simulink model "cl_e_5x"  (Simulink 7.4)
settings: Solver=ode15s  StartTime=0.0  StopTime=inf  MaxStep=5e-9  RelTol=1e-5
PreLoadFcn:
  | f=3.9e6; Cp=3.6e-9; Cx=3e-9;
undefined symbols (not defined in the file or in its folder): One, sided
libraries: powerlib x16, simulink x1, dspsnks4 x1, dsparch4 x1
settings Model: Creator=dbenson  LastModifiedBy=Dick
settings DataIOCC: SaveOutput=off  SaveTime=off  SignalLoggingName=sigsOut
settings OptimizationCC: BooleanDataType=off  InlineInvariantSignals=on  InitFltsAndDblsToZero=on
settings DebuggingCC: SaveWithParameterizedLinksMsg=none  SignalResolutionControl=TryResolveAllWithWarning  SolverPrmCheckMsg=none  MultiTaskDSMMsg=warning  MultiTaskCondExecSysMsg=none  StrictBusMsg=None
settings HardwareCC: TargetUnknown=on
settings RTWCC: IncludeERTFirstTime=on
settings GRTTargetCC: TargetFcnLib=ansi_tfl_tmw.mat

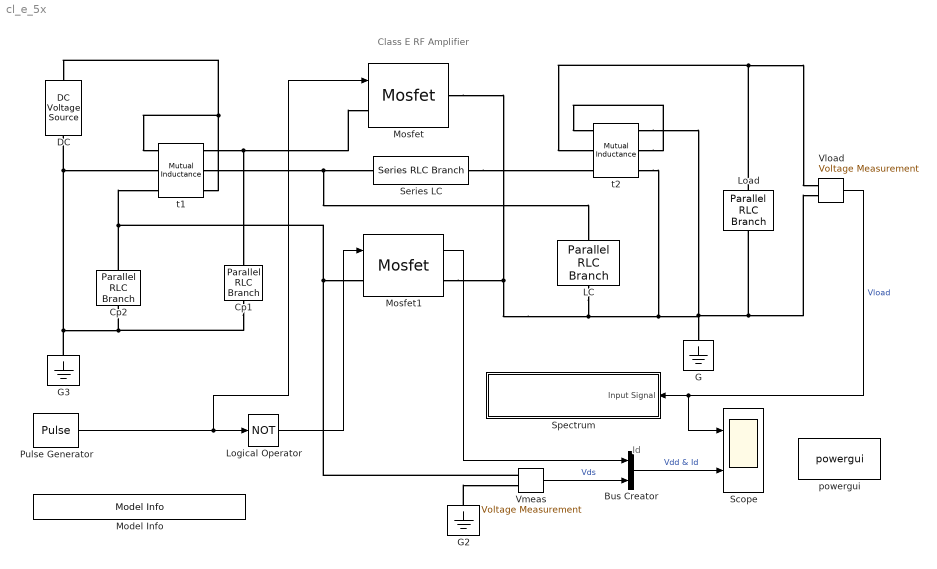
== system cl_e_5x ==
  note: Id
  note: Class E RF Amplifier
  Bus Creator : BusCreator  Inputs=2
  Cp1 : powerlib/Elements/Parallel RLC Branch  DialogController=POWERSYS.PowerSysDialog  PhysicalDomain=powersysdomain  SubClassName=unknown  LeftPortType=p1  RightPortType=p1  LConnTagsString=a  RConnTagsString=__new0  BranchType=C  Resistance=1.0  Inductance=1.0  SetiL0=off  InitialCurrent=0  Capacitance=Cp  Setx0=off  InitialVoltage=0  Measurements=None
  Cp2 : powerlib/Elements/Parallel RLC Branch  DialogController=POWERSYS.PowerSysDialog  PhysicalDomain=powersysdomain  SubClassName=unknown  LeftPortType=p1  RightPortType=p1  LConnTagsString=a  RConnTagsString=__new0  BranchType=C  Resistance=1.0  Inductance=1.0  SetiL0=off  InitialCurrent=0  Capacitance=Cp  Setx0=off  InitialVoltage=0  Measurements=None
  DC : powerlib/Electrical Sources/DC Voltage Source  Description=source block  DialogController=POWERSYS.PowerSysDialog  SystemSampleTime=-1  Amplitude=25  Measurements=None
      settings: AttributesFormatString=\n
  G : powerlib/Elements/Ground  DialogController=POWERSYS.PowerSysDialog  PhysicalDomain=powersysdomain  SubClassName=unknown  LeftPortType=p1  RightPortType=p1  LConnTagsString=a
  G2 : powerlib/Elements/Ground  DialogController=POWERSYS.PowerSysDialog  PhysicalDomain=powersysdomain  SubClassName=unknown  LeftPortType=p1  RightPortType=p1  LConnTagsString=a
  G3 : powerlib/Elements/Ground  DialogController=POWERSYS.PowerSysDialog  PhysicalDomain=powersysdomain  SubClassName=unknown  LeftPortType=p1  RightPortType=p1  LConnTagsString=a
  LC : powerlib/Elements/Parallel RLC Branch  DialogController=POWERSYS.PowerSysDialog  PhysicalDomain=powersysdomain  SubClassName=unknown  LeftPortType=p1  RightPortType=p1  LConnTagsString=a  RConnTagsString=__new0  BranchType=LC  Resistance=1.0  Inductance=1e-6  SetiL0=off  InitialCurrent=0  Capacitance=Cx  Setx0=off  InitialVoltage=0  Measurements=None
  Load : powerlib/Elements/Parallel RLC Branch  DialogController=POWERSYS.PowerSysDialog  PhysicalDomain=powersysdomain  SubClassName=unknown  LeftPortType=p1  RightPortType=p1  LConnTagsString=a  RConnTagsString=__new0  BranchType=RC  Resistance=50  Inductance=1.0  SetiL0=off  InitialCurrent=0  Capacitance=300e-12  Setx0=off  InitialVoltage=0  Measurements=None
  Logical Operator : Logic  Operator=NOT  AllPortsSameDT=off
  Model Info : simulink/Model-Wide Utilities/Model Info  SystemSampleTime=-1  InitialBlockCM=None  BlockCM=None  Frame=on  DisplayStringWithTags=Copywrite 2005-2010 The MathWorks, Inc.  HorizontalTextAlignment=Center  LeftAlignmentValue=0.5  SourceBlockDiagram=cl_e_5x  TagMaxNumber=20
  Mosfet : powerlib/Power Electronics/Mosfet  DialogController=POWERSYS.PowerSysDialog  SystemSampleTime=-1  Ron=1  Lon=150e-9  Rd=.001  Vfd=0  IC=0  Rs=0  Cs=0  Measurements=off
      settings: AttributesFormatString=\n
  Mosfet1 : powerlib/Power Electronics/Mosfet  DialogController=POWERSYS.PowerSysDialog  SystemSampleTime=-1  Ron=1  Lon=150e-9  Rd=.001  Vfd=0  IC=0  Rs=0  Cs=0  Measurements=on
      settings: AttributesFormatString=\n
  Pulse Generator : DiscretePulseGenerator  PulseType=Time based  Amplitude=2  Period=1/f  PulseWidth=50  PhaseDelay=0  SampleTime=1
  Scope : Scope  NumInputPorts=2
      settings: TimeRange=1.282051282051282e-006  YMin=-100~-30  YMax=100~80  MaxDataPoints=2000  SampleInput=on
  "Series LC " : powerlib/Elements/Series RLC Branch  DialogController=POWERSYS.PowerSysDialog  PhysicalDomain=powersysdomain  SubClassName=unknown  LeftPortType=p1  RightPortType=p1  LConnTagsString=__new0  RConnTagsString=__new0  BranchType=LC  Resistance=1.0  Inductance="4*1e-6  - 0.9e-6"  SetiL0=off  InitialCurrent=0  Capacitance=2.1e-9/4  Setx0=off  InitialVoltage=0  Measurements=None
  Spectrum : Subsystem  Description=Spectrum Analyzer  mask{BW=30e6, Zo=50}
      mask prompts: BW "Bandwidth"; Zo "Load Zo"
      mask Display: fprintf('Baseband Spectrum Analyzer \n  BW=%7.2f MHz', BW/1e6)
  Vload : powerlib/Measurements/Voltage Measurement  Tag=PoWeRsYsTeMmEaSuReMeNt  DialogController=POWERSYS.PowerSysDialog  SystemSampleTime=-1  PhasorSimulation=off  OutputType=Magnitude  PSBequivalent=0
  "Vmeas " : powerlib/Measurements/Voltage Measurement  Tag=PoWeRsYsTeMmEaSuReMeNt  DialogController=POWERSYS.PowerSysDialog  SystemSampleTime=-1  PhasorSimulation=off  OutputType=Magnitude  PSBequivalent=0
  powergui : powerlib/powergui  Priority=1  SystemSampleTime=-1  SimulationMode=Continuous  SampleTime=50e-6  frequency=60  SPID=off  DisableSnubberDevices=off  DisableRonSwitches=off  DisableVfSwitches=off  SwTol=0  Interpol=off  frequencyindice=0  echomessages=off  HookPort=off  DisplayEquations=off  FunctionMessages=off  EnableUseOfTLC=off  x0status=blocks  RestoreLinks=warning  Frange=[0:2:500]  Ylog=off  Xlog=on  ShowGrid=off  save=off  variable=ZData  ZoomFFT=on  StartTime=0.0  cycles=1  DisplayStyle=1  fundamental=60  FreqAxis=off  MaxFrequency=1000  frequencyindicesteady=1  RmsSteady=1  display=off  Ts=0  methode=off
  t1 : powerlib/Elements/Mutual Inductance  DialogController=POWERSYS.PowerSysDialog  PhysicalDomain=powersysdomain  SubClassName=unknown  LeftPortType=p1  RightPortType=p1  LConnTagsString=a|b|c  RConnTagsString=A|B|C  TypeOfMutual=Two or three windings with equal mutual terms  NumberOfWindings=3  SelfImpedance1=[0.1 1e-04 ]  SelfImpedance2=[ 0.1 1e-04]  ThreeWindings=on  SelfImpedance3=[ 0.1 1e-04]  MutualImpedance=[0.0 0.9999e-04]  InductanceMatrix="[1.0 0.9  0.9 ;  0.9 1.0  0.9;  0.9 0.9 1.0 ] * 1e-3"  ResistanceMatrix="[1.0 0.9  0.9 ;  0.9 1.0  0.9;  0.9 0.9 1.0 ]"  Measurements=None
      settings: AttributesFormatString=\n
  t2 : powerlib/Elements/Mutual Inductance  DialogController=POWERSYS.PowerSysDialog  PhysicalDomain=powersysdomain  SubClassName=unknown  LeftPortType=p1  RightPortType=p1  LConnTagsString=a|b|c  RConnTagsString=A|B|C  TypeOfMutual=Two or three windings with equal mutual terms  NumberOfWindings=3  SelfImpedance1=[0.1 1e-04 ]  SelfImpedance2=[ 0.1 1e-04]  ThreeWindings=on  SelfImpedance3=[ 0.1 1e-04]  MutualImpedance=[0.0 0.9999e-04]  InductanceMatrix="[1.0 0.9  0.9 ;  0.9 1.0  0.9;  0.9 0.9 1.0 ] * 1e-3"  ResistanceMatrix="[1.0 0.9  0.9 ;  0.9 1.0  0.9;  0.9 0.9 1.0 ]"  Measurements=None
      settings: AttributesFormatString=\n
  wires:
  Pulse Generator/1 -> Logical Operator/1, Mosfet/1
  Bus Creator/1 -> Scope/2  "Vdd & Id"
  "Vmeas "/1 -> Bus Creator/2  "Vds"
  Mosfet1/1 -> Bus Creator/1
  Vload/1 -> Scope/1, Spectrum/1(Input Signal)  "Vload"
  Logical Operator/1 -> Mosfet1/1
  connections:
  G3/LConn1 -- DC/LConn1 -- t1/LConn2 -- Cp2/LConn1 -- Cp1/RConn1
  "Series LC "/RConn1 -- t2/LConn3
  t2/RConn2 -- t2/LConn1
  t2/RConn1 -- G/LConn1 -- t2/RConn3 -- LC/RConn1 -- Mosfet1/RConn1 -- Mosfet/RConn1 -- Load/LConn1 -- Vload/LConn2
  t1/RConn2 -- "Series LC "/LConn1 -- LC/LConn1
  Load/RConn1 -- Vload/LConn1 -- t2/LConn2
  G2/LConn1 -- "Vmeas "/LConn2
  "Vmeas "/LConn1 -- Cp2/RConn1 -- t1/LConn3 -- Mosfet1/LConn1
  t1/RConn3 -- DC/RConn1 -- t1/LConn1
  t1/RConn1 -- Mosfet/LConn1 -- Cp1/LConn1

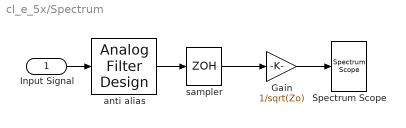
== system cl_e_5x/Spectrum ==
  Input Signal : Inport  OutDataType=sfix(16)  OutScaling=2^0
  Gain : Gain  Gain=1/sqrt(Zo)  ParameterDataType=fixdt(1, 16)  ParameterScaling=2^0  OutDataType=fixdt(1, 16)  OutScaling=2^0
  Spectrum Scope : dspsnks4/Spectrum Scope  DialogController=dspdialog.SpectrumScope  DialogControllerArgs=DataTag0  SystemSampleTime=-1  ScopeProperties=on  Domain=Frequency  HorizSpan=1  UseBuffer=on  BufferSize=512  Overlap=0  inpFftLenInherit=off  FFTlength=128  numAvg=1  DisplayProperties=off  AxisGrid=on  Memory=off  FrameNumber=on  AxisLegend=off  AxisZoom=off  OpenScopeAtSimStart=on  OpenScopeImmediately=off  FigPos=[575 32 408 280]  AxisProperties=off  XUnits=Hertz  XRange=One-sided ([0...Fs/2])  XDisplay=0  InheritXIncr=on  XIncr=1.0  XLabel=Samples  XLimit=Auto  YUnits=dBm  XMax=1  XMin=0  YLabel=dBm  LineProperties=off  wintypeSpecScope=Hann  RsSpecScope=50  betaSpecScope=5  winsampSpecScope=Periodic  XAxisParamsVer=6.9
      settings: YMin=-50  YMax=50
  anti alias : dsparch4/Analog Filter Design  method=Elliptic  filttype=Lowpass  N=8  Wlo=BW*2*pi  Whi=80  Rp=0.11  Rs=100
  sampler : ZeroOrderHold  SampleTime=1/(2.56*BW)
  wires:
  Gain/1 -> Spectrum Scope/1
  Input Signal/1 -> anti alias/1
  anti alias/1 -> sampler/1
  sampler/1 -> Gain/1
